simulink model "REI_s"  (R2021a)
settings: Solver=VariableStepAuto  StartTime=0.0  StopTime=100  RelTol=1e-3
values from neighbouring files (symbols this model uses):
  KUP = KsUP(1:4)    [REI.m]
libraries: cstblocks x5, simulink x1
settings Model: Creator=sofia  LastModifiedBy=sofia

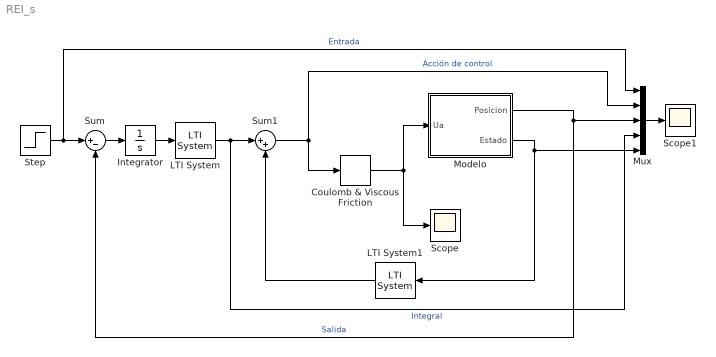
== system REI_s ==
  Coulomb & Viscous Friction : simulink/Discontinuities/Coulomb & Viscous Friction  offset=[0.4]  gain=1
  Integrator : Integrator
  LTI System : cstblocks/LTI System  sys=KiUP  IC=[]
  LTI System1 : cstblocks/LTI System  sys=-KUP  IC=[]
  Modelo : Subsystem
  Mux : Mux  Inputs=5
  Scope : Scope
  Scope1 : Scope
  Step : Step  After=0.5  SampleTime=0
  Sum : Sum  Inputs=|+-
  Sum1 : Sum  Inputs=|++
  wires:
  Step/1 -> Mux/1, Sum/1  "Entrada"
  Sum/1 -> Integrator/1
  Integrator/1 -> LTI System/1
  LTI System/1 -> Mux/4, Sum1/1  "Integral"
  Coulomb & Viscous Friction/1 -> Scope/1, Modelo/1(Ua)
  Sum1/1 -> Coulomb & Viscous Friction/1, Mux/2  "Acción de control"
  LTI System1/1 -> Sum1/2
  Modelo/2(Estado) -> LTI System1/1, Mux/5
  Modelo/1(Posicion) -> Mux/3, Sum/2  "Salida"
  Mux/1 -> Scope1/1

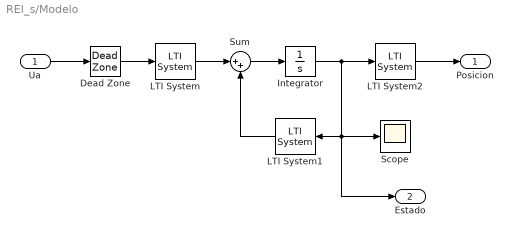
== system REI_s/Modelo ==
  Ua : Inport
  Dead Zone : DeadZone  UpperValue=0.6  SaturateOnIntegerOverflow=on
  Integrator : Integrator
  LTI System : cstblocks/LTI System  sys=B  IC=[]
  LTI System1 : cstblocks/LTI System  sys=A  IC=[]
  LTI System2 : cstblocks/LTI System  sys=C  IC=[]
  Scope : Scope
  Sum : Sum  Inputs=|++
  Posicion : Outport
  Estado : Outport  Port=2  PortDimensions=4
  wires:
  Integrator/1 -> LTI System2/1, Estado/1, Scope/1, LTI System1/1
  LTI System2/1 -> Posicion/1
  LTI System/1 -> Sum/1
  LTI System1/1 -> Sum/2
  Ua/1 -> Dead Zone/1
  Dead Zone/1 -> LTI System/1
  Sum/1 -> Integrator/1
